simulink model "ss_feedback"  (R2022a)
settings: Solver=VariableStepAuto  StartTime=0.0  StopTime=500  RelTol=1e-3
values from neighbouring files (symbols this model uses):
  A0 = [-3 1;-2 0]    [delayIndependent_analysis.m]    (also in delayIndependent_synthesis.m)
  A1 = [0 2]'    [delayIndependent_analysis.m]    (also in delayIndependent_synthesis.m)
  K = -[0.9 0]    [delayIndependent_analysis.m]    (also in delayIndependent_synthesis.m = Y*P)
settings Model: Creator=aaron  LastModifiedBy=aaron

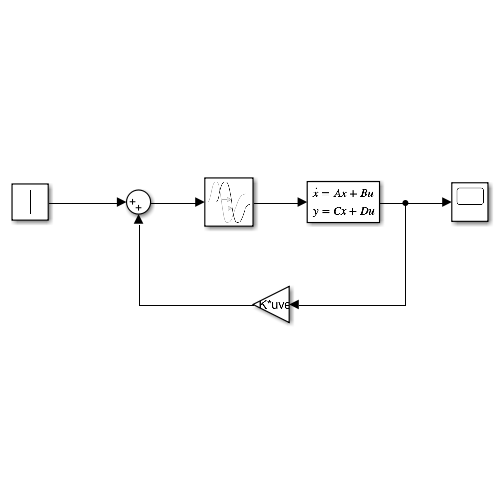
[thumbnail: Simulink's stored preview of the top-level diagram]
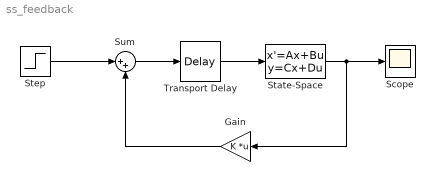
== system ss_feedback ==
  Gain : Gain  Gain=K  Multiplication=Matrix(K*u) (u vector)
  Scope : Scope
  State-Space : StateSpace  A=A0  B=A1  C=eye(2)  D=zeros(2,1)  InitialCondition=0
  Step : Step  Time=0  SampleTime=0
  Sum : Sum  Inputs=|++
  Transport Delay : TransportDelay  DelayTime=100
  wires:
  Transport Delay/1 -> State-Space/1
  Step/1 -> Sum/1
  Sum/1 -> Transport Delay/1
  Gain/1 -> Sum/2
  State-Space/1 -> Scope/1, Gain/1
